simulink model "anirban"  (R2021a)
settings: Solver=ode23tb  StartTime=0.0  StopTime=1000  RelTol=1e-3
libraries: pid_lib x1
settings Model: Creator=ITER  LastModifiedBy=Tapas
settings SolverCC: AlgebraicLoopSolver=TrustRegion
settings DebuggingCC: UnconnectedInputMsg=none  UnconnectedOutputMsg=none  UnconnectedLineMsg=none  SFMachineParentedDataDiag=warning  ArithmeticOperatorsInVariantConditions=warning
settings ModelReferenceCC: EnableRefExpFcnMdlSchedulingChecks=off
settings SFSimCC: CustomCodeUndefinedFunction=UseInterfaceOnly
settings RTWCC: Description=Generic Real-Time Target

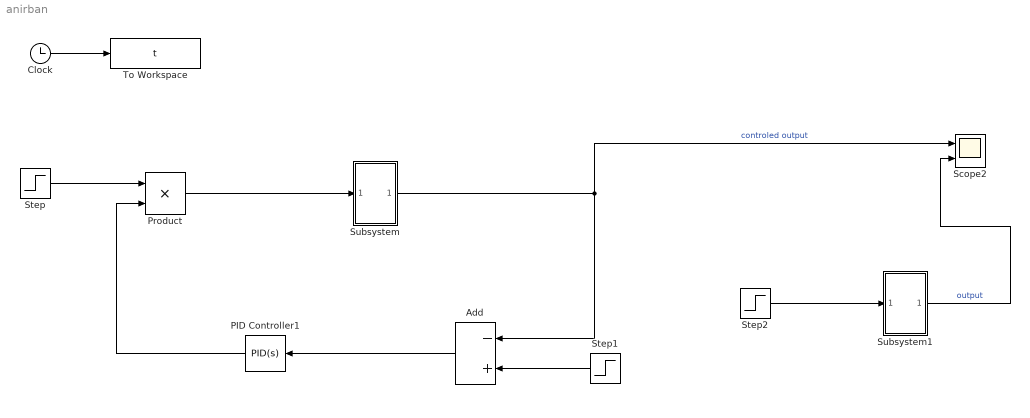
== system anirban ==
  Add : Sum  Inputs=-+
  Clock : Clock
  PID Controller1 : pid_lib/PID Controller  Controller=PID  Form=Parallel  TimeDomain=Continuous-time  UseExternalTs=off  SampleTime=-1  IntegratorMethod=Forward Euler  FilterMethod=Forward Euler  ControllerParametersSource=internal  P=0  I=0.00316628398292372  D=0  UseFilter=on  N=100  TunerSelectOption=Transfer Function Based (PID Tuner App)  InitialConditionSource=internal  InitialConditionForIntegrator=0  InitialConditionForFilter=0  DifferentiatorICPrevScaledInput=0  ExternalReset=none  TrackingMode=off  Kt=1  LimitOutput=off  SatLimitsSource=internal  UpperSaturationLimit=inf  LowerSaturationLimit=-inf  LinearizeAsGain=on  AntiWindupMode=none  Kb=1  POutMin=[]  POutMax=[]  IOutMin=[]  IOutMax=[]  DOutMin=[]  DOutMax=[]  NOutMin=[]  NOutMax=[]  SumOutMin=[]  SumOutMax=[]  SaturationOutMin=[]  SaturationOutMax=[]  PParamMin=[]  PParamMax=[]  IParamMin=[]  IParamMax=[]  DParamMin=[]  DParamMax=[]  NParamMin=[]  NParamMax=[]  KbParamMin=[]  KbParamMax=[]  KtParamMin=[]  KtParamMax=[]  KbOutMin=[]  KbOutMax=[]  KtOutMin=[]  KtOutMax=[]  IntegratorOutMin=[]  IntegratorOutMax=[]  FilterOutMin=[]  FilterOutMax=[]  SumI1OutMin=[]  SumI1OutMax=[]  SumI2OutMin=[]  SumI2OutMax=[]  SumI3OutMin=[]  SumI3OutMax=[]  SumI4OutMin=[]  SumI4OutMax=[]  SumDOutMin=[]  SumDOutMax=[]  DifferentiatorOutMin=[]  DifferentiatorOutMax=[]  FilterDiffOutCoefMin=[]  FilterDiffOutCoefMax=[]  ReciprocalOutMin=[]  ReciprocalOutMax=[]  SumDenOutMin=[]  SumDenOutMax=[]  SumNumOutMin=[]  SumNumOutMax=[]  DivideOutMin=[]  DivideOutMax=[]  UdiffTsProdOutMin=[]  UdiffTsProdOutMax=[]  NTsProdOutMin=[]  NTsProdOutMax=[]  UintegralTsProdOutMin=[]  UintegralTsProdOutMax=[]  UngainTsProdOutMin=[]  UngainTsProdOutMax=[]  IntegratorContinuousStateAttributes=''  IntegratorStateMustResolveToSignalObject=off  IntegratorRTWStateStorageClass=Auto  FilterContinuousStateAttributes=''  FilterStateMustResolveToSignalObject=off  FilterRTWStateStorageClass=Auto  ParallelPVariant=InternalParameters  IdealPVariant=Disabled  IVariant=InternalParameters  DVariant=InternalParameters  IntegratorVariant=Continuous  SatVariant=Disabled  AWVariant=Passthrough  PCopyVariant=Disabled  TRVariant=Disabled  FdbkBlocksVariant=Forward  IdealPFdbkVariant=Disabled  SatFdbkVariant=Disabled  DerivativeFilterVariant=ContFilter  NVariant=InternalParameters  NCopyVariant=Disabled  FilterICVariant=InternalICsFilter  IntegratorICVariant=InternalICs  ExternalResetVariant=Disabled  TRSumVariant=Passthrough  SumFdbkVariant=Disabled  SumVariant=Sum_PID  TsampFilterVariant=InternalTs  TsampNgainVariant=Passthrough  TsampIntegralVariant=Passthrough  ExternalSaturationOutDataTypeStr=Inherit: Same as second input
  Product : Product
  Scope2 : Scope  NumInputPorts=2
  Step : Step  Time=0  After=10  SampleTime=0
  Step1 : Step  Time=0  After=4  SampleTime=0
  Step2 : Step  Time=0  After=10  SampleTime=0
  Subsystem : Subsystem
  Subsystem1 : Subsystem
  To Workspace : ToWorkspace  VariableName=t  SaveFormat=Timeseries  SampleTime=-1
  wires:
  Subsystem/1(Out1) -> Add/1, Scope2/1  "controled output"
  Step/1 -> Product/1
  PID Controller1/1 -> Product/2
  Add/1 -> PID Controller1/1
  Step1/1 -> Add/2
  Product/1 -> Subsystem/1(In1)
  Clock/1 -> To Workspace/1
  Step2/1 -> Subsystem1/1(In1)
  Subsystem1/1(Out1) -> Scope2/2  "output"

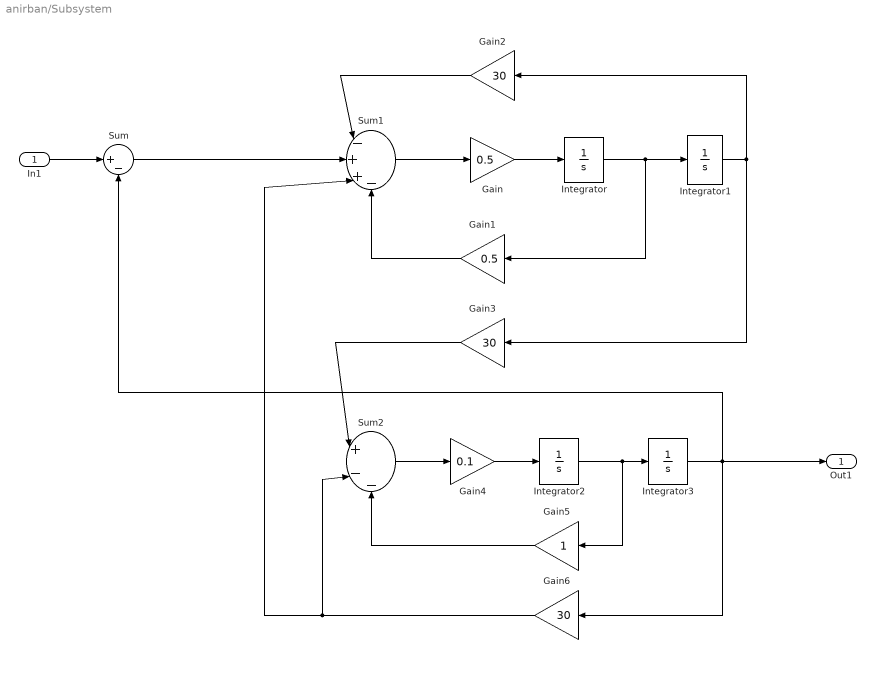
== system anirban/Subsystem ==
  In1 : Inport
  Gain : Gain  Gain=0.5
  Gain1 : Gain  Gain=0.5
  Gain2 : Gain  Gain=30
  Gain3 : Gain  Gain=30
  Gain4 : Gain  Gain=0.1
  Gain5 : Gain
  Gain6 : Gain  Gain=30
  Integrator{,1..3} (4 alike) : Integrator
  Sum : Sum  Inputs=|+-
  Sum1 : Sum  Inputs=|-++-
  Sum2 : Sum  Inputs=|+--
  Out1 : Outport
  wires:
  Gain6/1 -> Sum2/2, Sum1/3
  Sum/1 -> Sum1/2
  Integrator2/1 -> Gain5/1, Integrator3/1
  Gain4/1 -> Integrator2/1
  Integrator/1 -> Gain1/1, Integrator1/1
  Gain5/1 -> Sum2/3
  Integrator3/1 -> Out1/1, Sum/2, Gain6/1
  Integrator1/1 -> Gain2/1, Gain3/1
  Gain1/1 -> Sum1/4
  Sum2/1 -> Gain4/1
  Gain2/1 -> Sum1/1
  Gain/1 -> Integrator/1
  Sum1/1 -> Gain/1
  Gain3/1 -> Sum2/1
  In1/1 -> Sum/1

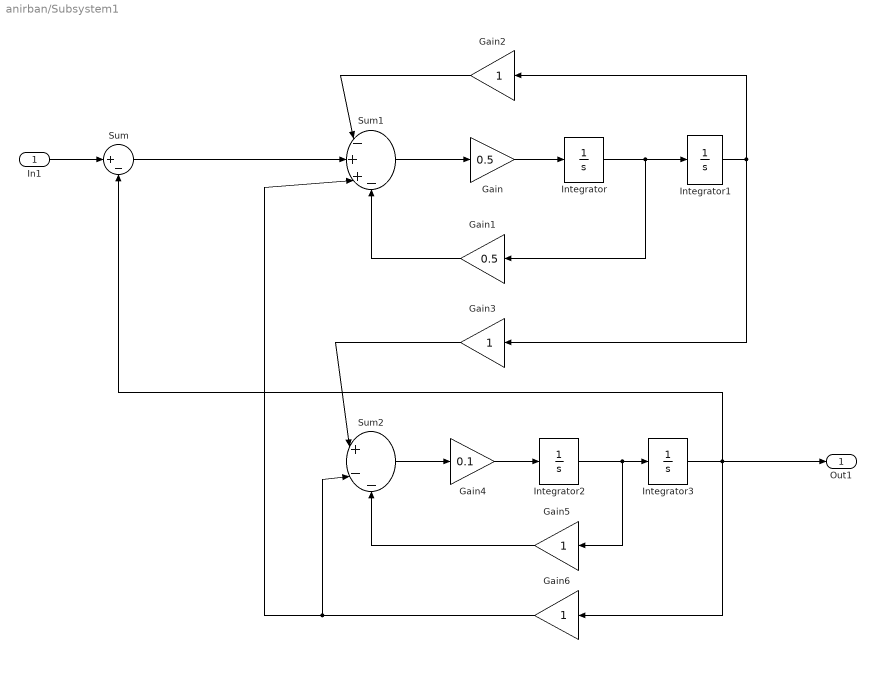
== system anirban/Subsystem1 ==
  In1 : Inport
  Gain : Gain  Gain=0.5
  Gain1 : Gain  Gain=0.5
  Gain{2..3,5..6} (4 alike) : Gain
  Gain4 : Gain  Gain=0.1
  Integrator{,1..3} (4 alike) : Integrator
  Sum : Sum  Inputs=|+-
  Sum1 : Sum  Inputs=|-++-
  Sum2 : Sum  Inputs=|+--
  Out1 : Outport
  wires:
  Gain6/1 -> Sum2/2, Sum1/3
  Sum/1 -> Sum1/2
  Integrator2/1 -> Gain5/1, Integrator3/1
  Gain4/1 -> Integrator2/1
  Integrator/1 -> Gain1/1, Integrator1/1
  Gain5/1 -> Sum2/3
  Integrator3/1 -> Out1/1, Sum/2, Gain6/1
  Integrator1/1 -> Gain2/1, Gain3/1
  Gain1/1 -> Sum1/4
  Sum2/1 -> Gain4/1
  Gain2/1 -> Sum1/1
  Gain/1 -> Integrator/1
  Sum1/1 -> Gain/1
  Gain3/1 -> Sum2/1
  In1/1 -> Sum/1
